simulink model "MBDques1_1"  (R2020a)
settings: Solver=VariableStepAuto  StartTime=0.0  StopTime=10.0  RelTol=1e-3
undefined symbols (not defined in the file): b, k1, k12, M1
settings Model: Creator=DELL  LastModifiedBy=DELL

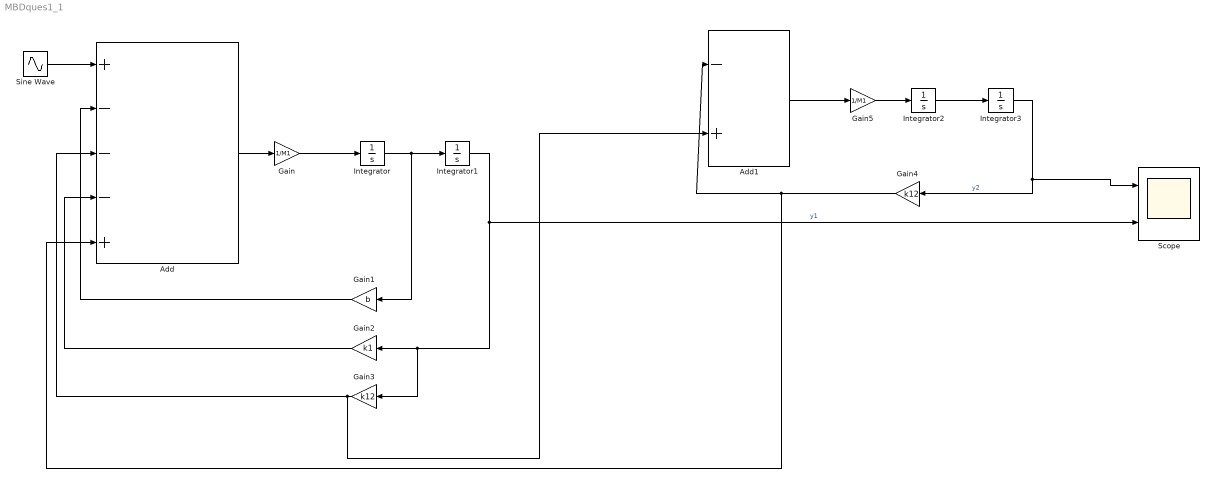
== system MBDques1_1 ==
  Add : Sum  Inputs=+---+
  Add1 : Sum  Inputs=-+
  Gain : Gain  Gain=1/M1
  Gain1 : Gain  Gain=b
  Gain2 : Gain  Gain=k1
  Gain3 : Gain  Gain=k12
  Gain4 : Gain  Gain=k12
  Gain5 : Gain  Gain=1/M1
  Integrator{,1..3} (4 alike) : Integrator
  Scope : Scope  NumInputPorts=2
  Sine Wave : Sin  SampleTime=0
  wires:
  Add/1 -> Gain/1
  Integrator/1 -> Gain1/1, Integrator1/1
  Gain/1 -> Integrator/1
  Integrator1/1 -> Gain3/1, Gain2/1, Scope/2  "y1"
  Sine Wave/1 -> Add/1
  Gain1/1 -> Add/2
  Gain2/1 -> Add/4
  Gain3/1 -> Add/3, Add1/2
  Gain4/1 -> Add/5, Add1/1
  Add1/1 -> Gain5/1
  Integrator3/1 -> Scope/1, Gain4/1  "y2"
  Gain5/1 -> Integrator2/1
  Integrator2/1 -> Integrator3/1
